simulink model "hydrulictest"  (R2021a)
settings: Solver=VariableStepAuto  StartTime=0.0  StopTime=10.0  RelTol=1e-3
libraries: sh_lib x8, fl_lib x7, nesl_utility x7
settings Model: Creator=top10  LastModifiedBy=top10

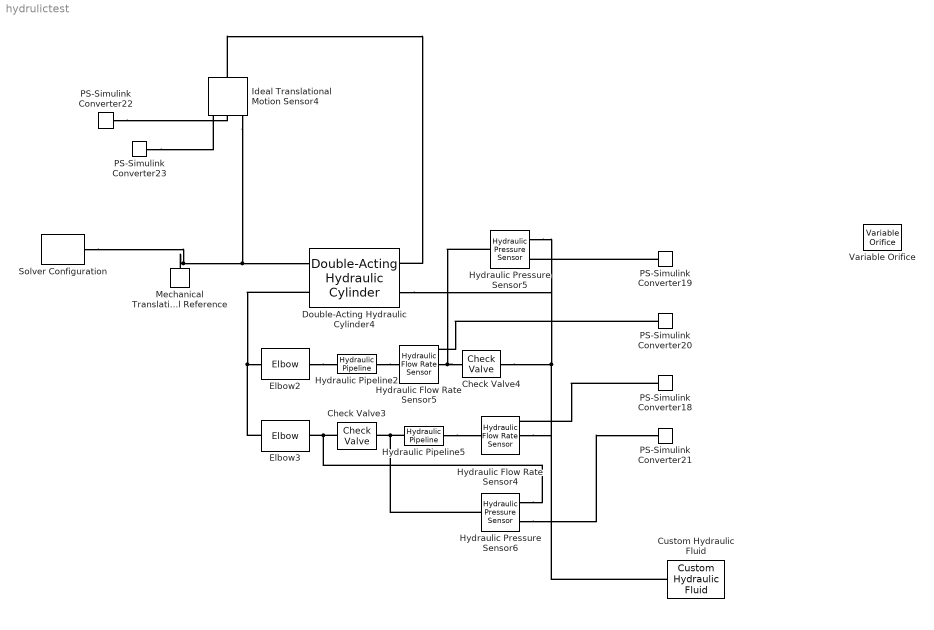
== system hydrulictest ==
  Check Valve3 : sh_lib/Valves/Directional Valves/Check Valve  area_max=1e-4 m^2  pres_crack=0.3e5 Pa  pres_max=1.2e5 Pa  C_d=0.7  A_leak=1e-12 m^2  lam_spec=1  B_lam=0.999  Re_cr=12  dynamic=0  tau=0.1 s  area_init=1e-12 m^2
      settings: SourceProductBaseCode=SH  InternalSimscapePortConfiguration="{\"Bottom\":[],\"Left\":[{\"id\":\"A\",\"label\":\"A\",\"type\":\"foundation.hydraulic.hydraulic\"}],\"Right\":[{\"id\":\"B\",\"label\":\"B\",\"type\":\"foundation.hydraulic.hydraulic\"}],\"Top\":[]}"
  Check Valve4 : sh_lib/Valves/Directional Valves/Check Valve  area_max=1e-4 m^2  pres_crack=0.3e5 Pa  pres_max=1.2e5 Pa  C_d=0.7  A_leak=1e-12 m^2  lam_spec=1  B_lam=0.999  Re_cr=12  dynamic=0  tau=0.1 s  area_init=1e-12 m^2
      settings: SourceProductBaseCode=SH  InternalSimscapePortConfiguration="{\"Bottom\":[],\"Left\":[{\"id\":\"A\",\"label\":\"A\",\"type\":\"foundation.hydraulic.hydraulic\"}],\"Right\":[{\"id\":\"B\",\"label\":\"B\",\"type\":\"foundation.hydraulic.hydraulic\"}],\"Top\":[]}"
  Custom Hydraulic Fluid : fl_lib/Hydraulic/Hydraulic Utilities/Custom Hydraulic Fluid  density=874 kg/m^3  viscosity_kin=46e-6 m^2/s  bulk=0.8e9 Pa  alpha=0.005  range_error=2
      settings: SourceProductBaseCode=SS  InternalSimscapePortConfiguration="{\"Bottom\":[],\"Left\":[],\"Right\":[{\"id\":\"G\",\"label\":\"\",\"type\":\"foundation.hydraulic.hydraulic\"}],\"Top\":[]}"
  Double-Acting Hydraulic Cylinder4 : sh_lib/Hydraulic Cylinders/Double-Acting Hydraulic Cylinder  area_A=a1 mm^2  area_B=a2 mm^2  stroke=stroke mm  dead_vol_A=1e-4 m^3  dead_vol_B=1e-4 m^3  k_sh=1.4  or=sh.cylinders.enum.MechOrientationTranslational.Positive  stiff=1e9 N/m  D=150 N/(m/s)  hardstop_model=1  transition=0.1 mm  displacement_spec=foundation.enum.DisplacementSpec.Calculate  init_pos=30 mm  init_pressure_A=0 Pa  init_pressure_B=0 Pa
      settings: SourceProductBaseCode=SH  InternalSimscapePortConfiguration="{\"Bottom\":[],\"Left\":[{\"id\":\"C\",\"label\":\"C\",\"type\":\"foundation.mechanical.translational.translational\"},{\"id\":\"A\",\"label\":\"A\",\"type\":\"foundation.hydraulic.hydraulic\"}],\"Right\":[{\"id\":\"R\",\"label\":\"R\",\"type\":\"foundation.mechanical.translational.translational\"},{\"id\":\"B\",\"label\":\"B\",\"type\":\"foundation.hydraulic.hydraulic\"}],\"Top\":[]}"
  Elbow2 : sh_lib/Local Hydraulic Resistances/Elbow  elbow_type=1  elbow_diam=p mm  elbow_angle=90 deg  lam_spec=1  B_lam=0.999  Re_cr=80
      settings: SourceProductBaseCode=SH  InternalSimscapePortConfiguration="{\"Bottom\":[],\"Left\":[{\"id\":\"A\",\"label\":\"A\",\"type\":\"foundation.hydraulic.hydraulic\"}],\"Right\":[{\"id\":\"B\",\"label\":\"B\",\"type\":\"foundation.hydraulic.hydraulic\"}],\"Top\":[]}"
  Elbow3 : sh_lib/Local Hydraulic Resistances/Elbow  elbow_type=1  elbow_diam=p mm  elbow_angle=90 deg  lam_spec=1  B_lam=0.999  Re_cr=80
      settings: SourceProductBaseCode=SH  InternalSimscapePortConfiguration="{\"Bottom\":[],\"Left\":[{\"id\":\"A\",\"label\":\"A\",\"type\":\"foundation.hydraulic.hydraulic\"}],\"Right\":[{\"id\":\"B\",\"label\":\"B\",\"type\":\"foundation.hydraulic.hydraulic\"}],\"Top\":[]}"
  Hydraulic Flow Rate Sensor4 : fl_lib/Hydraulic/Hydraulic Sensors/Hydraulic Flow Rate Sensor
  Hydraulic Flow Rate Sensor5 : fl_lib/Hydraulic/Hydraulic Sensors/Hydraulic Flow Rate Sensor
  Hydraulic Pipeline2 : sh_lib/Pipelines/Hydraulic Pipeline  cs_type=foundation.enum.pipeCrossSection.circular  d_in=p mm  area=1e-4 m^2  D_h=1.12e-2 m  s_factor=64  length=p_1 mm  length_ad=1 m  roughness=15e-6 m  Re_lam=2000  Re_turb=4000  wall_type=foundation.enum.chamber_spec.rigid  pr_r_coef=2e-12 m/Pa  time_const=0.01 s  k_sh=1.4  initial_pressure=0 Pa
      settings: SourceProductBaseCode=SH  InternalSimscapePortConfiguration="{\"Bottom\":[],\"Left\":[{\"id\":\"A\",\"label\":\"A\",\"type\":\"foundation.hydraulic.hydraulic\"}],\"Right\":[{\"id\":\"B\",\"label\":\"B\",\"type\":\"foundation.hydraulic.hydraulic\"}],\"Top\":[]}"
  Hydraulic Pipeline5 : sh_lib/Pipelines/Hydraulic Pipeline  cs_type=foundation.enum.pipeCrossSection.circular  d_in=p mm  area=1e-4 m^2  D_h=1.12e-2 m  s_factor=64  length=p_2 mm  length_ad=1 m  roughness=15e-6 m  Re_lam=2000  Re_turb=4000  wall_type=foundation.enum.chamber_spec.rigid  pr_r_coef=2e-12 m/Pa  time_const=0.01 s  k_sh=1.4  initial_pressure=0 Pa
      settings: SourceProductBaseCode=SH  InternalSimscapePortConfiguration="{\"Bottom\":[],\"Left\":[{\"id\":\"A\",\"label\":\"A\",\"type\":\"foundation.hydraulic.hydraulic\"}],\"Right\":[{\"id\":\"B\",\"label\":\"B\",\"type\":\"foundation.hydraulic.hydraulic\"}],\"Top\":[]}"
  Hydraulic Pressure Sensor5 : fl_lib/Hydraulic/Hydraulic Sensors/Hydraulic Pressure Sensor
  Hydraulic Pressure Sensor6 : fl_lib/Hydraulic/Hydraulic Sensors/Hydraulic Pressure Sensor
  Ideal Translational Motion Sensor4 : fl_lib/Mechanical/Mechanical Sensors/Ideal Translational Motion Sensor  offset=0 m
  Mechanical Translational Reference : fl_lib/Mechanical/Translational Elements/Mechanical Translational Reference
  PS-Simulink Converter{18..23} (6 alike) : nesl_utility/PS-Simulink Converter  PhysicalDomain=network_engine_domain  SubClassName=ps_output  LeftPortType=input  RightPortType=output  PseudoPeriodic=off  Frequencies=[]  Unit=inherit  AffineConversion=off
      settings: SourceProductBaseCode=PW,SS
  Solver Configuration : nesl_utility/Solver Configuration  PhysicalDomain=network_engine_domain  SubClassName=solver  LeftPortType=input  RightPortType=generic  Tones=[]  Harmonics=[]  SimulateNoise=off  Profile=off  UseLocalSampling=off  EnableSwitchedLinearOptims=on  FrequencyDomain=off  UseCCode=off  RelTol=0.001  AbsTol=1e-06  MinStep=1e-09  ToWorkspace=off  RevertToSquareIcSolve=off  NumHomotopyIterations=100  PhasorMode=off  PhasorModeNumHarmonics=1  DoDC=off  ResidualTolerance=1e-09  UseLocalSolver=off  LocalSolverChoice=NE_BACKWARD_EULER_ADVANCER  LocalSolverSampleTime=0.001  DoFixedCost=off  MaxNonlinIter=3  MaxModeIter=2  ComputeImpulses=off  ImpulseIterations=2  LinearAlgebra=auto  EquationFormulation=NE_TIME_EF  DelaysMemoryBudget=1024  AutomaticFiltering=on  FilteringTimeConstant=0.001  PartitionStorageMethod=AS_NEEDED  PartitionMemoryBudget=1024  PartitionMethod=ROBUST
      settings: SourceProductBaseCode=PW,SS
  Variable Orifice : sh_lib/Orifices/Variable Orifice  mdl_type=2  area_max=0.5e-4 m^2  opening_max=5e-3 m  opening_tab=Valve.angle mm  area_tab=Valve.orfice mm^2  pressure_tab=[-10000000, -5000000, -2000000, 2000000, 5000000, 10000000] Pa  flow_rate_tab=[-1e-07, -7.0711e-08, -4.4721e-08, 4.4721e-08, 7.0711e-08, 1e-07; -2.0352e-05, -1.4391e-05, -9.1017e-06, 9.1017e-06, 1.4391e-05, 2.0352e-05; -.0040736, -.0028805, -.0018218, .0018218, .0028805, .0040736; -.011438, -.0080879, -.0051152, .0051152, .0080879, .011438; -.034356, -.024293, -.015364, .015364, .024293, .034356] m^3/s  interp_method=1  extrap_method=1  or=1  C_d=0.7  x_0=0 m  A_leak=1e-12 m^2  lam_spec=1  B_lam=0.999  Re_cr=12  flow_rate_specify=off  flow_rate_priority=None  flow_rate=0 m^3/s  flow_rate_nominal_specify=off  flow_rate_nominal_unit=m^3/s  flow_rate_nominal_value=1  pressure_drop_specify=off  pressure_drop_priority=None  pressure_drop=0 Pa  pressure_drop_nominal_specify=off  pressure_drop_nominal_unit=Pa  pressure_drop_nominal_value=1
      settings: SourceProductBaseCode=SH  InternalSimscapePortConfiguration="{\"Bottom\":[],\"Left\":[{\"id\":\"S\",\"label\":\"S\",\"type\":\"input\"},{\"id\":\"A\",\"label\":\"A\",\"type\":\"foundation.hydraulic.hydraulic\"}],\"Right\":[{\"id\":\"B\",\"label\":\"B\",\"type\":\"foundation.hydraulic.hydraulic\"}],\"Top\":[]}"
  connections:
  Ideal Translational Motion Sensor4/LConn1 -- Double-Acting Hydraulic Cylinder4/RConn1
  Elbow3/LConn1 -- Elbow2/LConn1 -- Double-Acting Hydraulic Cylinder4/LConn2
  Check Valve3/LConn1 -- Hydraulic Pipeline5/LConn1 -- Hydraulic Pressure Sensor6/LConn1
  Check Valve4/RConn1 -- Custom Hydraulic Fluid/RConn1 -- Hydraulic Flow Rate Sensor4/RConn2 -- Double-Acting Hydraulic Cylinder4/RConn2 -- Hydraulic Pressure Sensor5/RConn1
  Hydraulic Pressure Sensor5/LConn1 -- Check Valve4/LConn1 -- Hydraulic Flow Rate Sensor5/RConn2
  Elbow3/RConn1 -- Check Valve3/RConn1 -- Hydraulic Pressure Sensor6/RConn1
  Mechanical Translational Reference/LConn1 -- Solver Configuration/RConn1 -- Ideal Translational Motion Sensor4/RConn1 -- Double-Acting Hydraulic Cylinder4/LConn1
  Hydraulic Pipeline2/RConn1 -- Hydraulic Flow Rate Sensor5/LConn1
  PS-Simulink Converter22/LConn1 -- Ideal Translational Motion Sensor4/RConn2
  PS-Simulink Converter23/LConn1 -- Ideal Translational Motion Sensor4/RConn3
  Hydraulic Pipeline5/RConn1 -- Hydraulic Flow Rate Sensor4/LConn1
  Hydraulic Pressure Sensor6/RConn2 -- PS-Simulink Converter21/LConn1
  Elbow2/RConn1 -- Hydraulic Pipeline2/LConn1
  PS-Simulink Converter18/LConn1 -- Hydraulic Flow Rate Sensor4/RConn1
  PS-Simulink Converter19/LConn1 -- Hydraulic Pressure Sensor5/RConn2
  PS-Simulink Converter20/LConn1 -- Hydraulic Flow Rate Sensor5/RConn1
